simulink model "sldrtex_model"  (R2020a)
settings: Solver=FixedStepAuto  StartTime=0.0  StopTime=600  RelTol=1e-3  EnableMultiTasking=on
settings Model: Creator=Ben  LastModifiedBy=Ben
settings SolverCC: AutoInsertRateTranBlk=on
settings DataIOCC: SaveFormat=StructureWithTime
settings OptimizationCC: BlockReduction=off  OptimizeBlockIOStorage=off
settings RTWCC: Description=Simulink Desktop Real-Time  SystemTargetFile=sldrt.tlc  TemplateMakefile=sldrt.tmf  RTWCompilerOptimization=on
settings CodeAppCC: MaxIdLength=95
settings SimulinkDesktopRealTimeCC: TargetPreCompLibLocation=C:\Program Files\MATLAB\R2020a\toolbox\sldrt\lib\win64  TargetLangStandard=C89/C90 (ANSI)

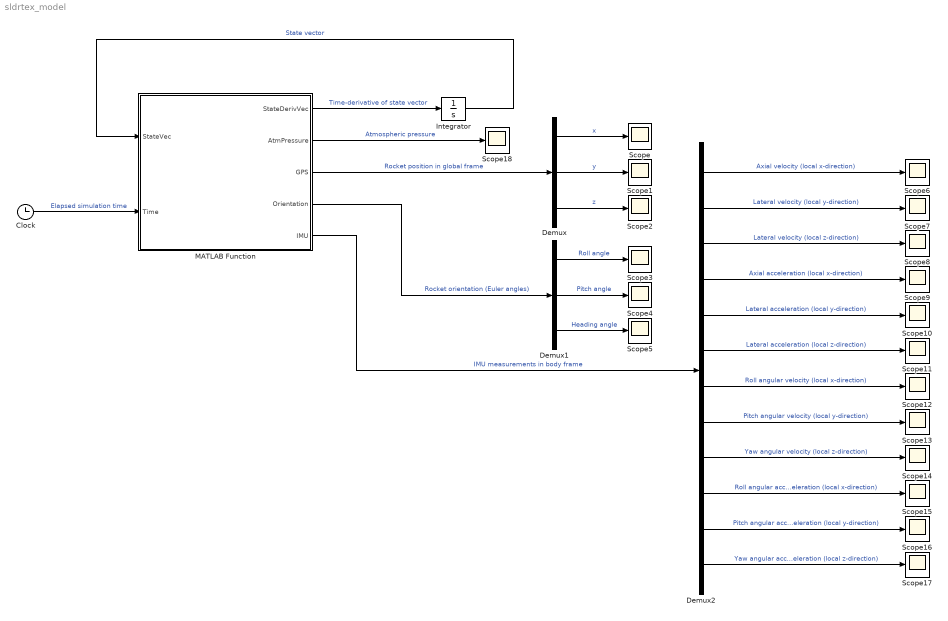
== system sldrtex_model ==
  Clock : Clock
  Demux : Demux  Outputs=3
  Demux1 : Demux  Outputs=3
  Demux2 : Demux  Outputs=12
  Integrator : Integrator  InitialCondition=[0 0 1401 0 -89 0 0 0 0 0 0 0]'
  MATLAB Function : MATLAB Function  TreatAsAtomicUnit=on
  Scope{,1..18} (19 alike) : Scope
  wires:
  Integrator/1 -> MATLAB Function/1(StateVec)  "State vector"
  MATLAB Function/1(StateDerivVec) -> Integrator/1  "Time-derivative of state vector"
  Clock/1 -> MATLAB Function/2(Time)  "Elapsed simulation time"
  MATLAB Function/2(AtmPressure) -> Scope18/1  "Atmospheric pressure"
  MATLAB Function/3(GPS) -> Demux/1  "Rocket position in global frame"
  MATLAB Function/4(Orientation) -> Demux1/1  "Rocket orientation (Euler angles)"
  MATLAB Function/5(IMU) -> Demux2/1  "IMU measurements in body frame"
  Demux/1 -> Scope/1  "x"
  Demux/2 -> Scope1/1  "y"
  Demux/3 -> Scope2/1  "z"
  Demux1/1 -> Scope3/1  "Roll angle"
  Demux1/3 -> Scope5/1  "Heading angle"
  Demux1/2 -> Scope4/1  "Pitch angle"
  Demux2/1 -> Scope6/1  "Axial velocity (local x-direction)"
  Demux2/2 -> Scope7/1  "Lateral velocity (local y-direction)"
  Demux2/3 -> Scope8/1  "Lateral velocity (local z-direction)"
  Demux2/4 -> Scope9/1  "Axial acceleration (local x-direction)"
  Demux2/7 -> Scope12/1  "Roll angular velocity (local x-direction)"
  Demux2/5 -> Scope10/1  "Lateral acceleration (local y-direction)"
  Demux2/8 -> Scope13/1  "Pitch angular velocity (local y-direction)"
  Demux2/6 -> Scope11/1  "Lateral acceleration (local z-direction)"
  Demux2/11 -> Scope16/1  "Pitch angular acceleration (local y-direction)"
  Demux2/9 -> Scope14/1  "Yaw angular velocity (local z-direction)"
  Demux2/12 -> Scope17/1  "Yaw angular acceleration (local z-direction)"
  Demux2/10 -> Scope15/1  "Roll angular acceleration (local x-direction)"

== matlab function sldrtex_model/MATLAB Function ==
  data: StateVec input double size=12,1; StateDerivVec output double size=12,1; Time input double size=1,1; AtmPressure output double size=1,1; GPS output double size=3,1; Orientation output double size=3,1; IMU output double size=12,1
function [StateDerivVec,AtmPressure,GPS,Orientation,IMU] = RocketDynModel_Sim(StateVec,Time)
%% Extract states and inputs
% States
PosVec = StateVec(1:3);
RollAngle = StateVec(4);
ElevAngle = StateVec(5);
HeadAngle = StateVec(6);
VelVec = StateVec(7:9);
AngVelVec_B = StateVec(10:12);

%% Define parameters
% Global properties
EarthRad = 6371.009e3;
GravAccelSL = 9.81;
WindVelVec = [0 0 0]';
SpHeatRatio = 1.4;

% Rocket physical properties
BurnTime = 34;
LoadMass = 711.9440829;
FuseDia = 0.508;
FuseLength = 7.90936;
PropFlowRate = 12.5;
NozzleEff = 0.98;
C_Star = 1580.684648;
ExitPressure = 78522.89615;
ChamberPressure = 950000;
ExpAreaRatio = 2.5;

% Rocket drag properties
P = load('Rocket drag data.mat');
MachNumData = P.RocketDragData(:,1);
DragCoeffData = P.RocketDragData(:,2);
DragArea = pi/4*FuseDia^2;
ACRelBasePosVec_B = [0.625 0 0]';
DirVec_B = [1 0 0]';

% Rocket launch properties
LaunchAngle = 89;
if Time <= 0
    if ElevAngle ~= -LaunchAngle
        error('Launch angle does not match initial elevation angle...');
    end
end
InitDistAlongRail = 0;
LaunchAlt = 1401;
RailLength = 15;
RailFricCoeff = 0;
LaunchVec = [
 cosd(LaunchAngle);
 0;
 sind(LaunchAngle)];

% Chute properties
BalluteAlt = 75000;
MainChuteAlt = 3000;
BalluteDragCoeff = 0.75;
MainChuteDragCoeff = 0.53;
BalluteLineLength = 5;
MainChuteLineLength = 7.148;
BalluteDia = 1;
MainChuteDia = 4.13;
NumBallutes = 3;
NumMainChutes = 3;
BalluteArea = NumBallutes*pi/4*(BalluteDia^2);
MainChuteArea = NumMainChutes*pi/4*(MainChuteDia^2);
ChuteRelBasePosVec_B = [5.66 0 0]';

% Rocket interial properties
Mass = ComputeRocketMass(Time,BurnTime,LoadMass,PropFlowRate);
[CGRelBasePosVec_B,CGRelBaseVelVec_B,CGRelBaseAccVec_B] =...
 ComputeCGRelBase(Time,BurnTime);
MOIMat = [ % Fix this to account for non-centered CG along cylinder
 (1/2)*Mass*(FuseDia/2)^2 0 0;
 0 (1/12)*Mass*(3*(FuseDia/2)^2 + FuseLength^2) 0;
 0 0 (1/12)*Mass*(3*(FuseDia/2)^2 + FuseLength^2)];
[AirDensity,SoundSpeed,~,AtmPressure,~,~,~] = atmos(PosVec(3),0,[],'SI','geometric',false);
GravAccel = GravAccelSL*((EarthRad/(EarthRad + PosVec(3)))^2);

%% Kinematics
% Fuselage rotation matrices
HeadRotMat = [
 cosd(HeadAngle) -sind(HeadAngle) 0;
 sind(HeadAngle) cosd(HeadAngle) 0;
 0 0 1];
ElevRotMat = [
 cosd(ElevAngle) 0 sind(ElevAngle);
 0 1 0;
 -sind(ElevAngle) 0 cosd(ElevAngle)];
RollRotMat = [
 1 0 0;
 0 cosd(RollAngle) -sind(RollAngle);
 0 sind(RollAngle) cosd(RollAngle)];
TotalRotMat = HeadRotMat*ElevRotMat*RollRotMat;

% Euler angle matrices
EulerRotMat = [
 1 0 -sind(ElevAngle);
 0 cosd(RollAngle) cosd(ElevAngle)*sind(RollAngle);
 0 -sind(RollAngle) cosd(ElevAngle)*cosd(RollAngle)];

% Forward coordinate transformation matrices
HeadTransMat_F = HeadRotMat';
ElevTransMat_F = ElevRotMat';
RollTransMat_F = RollRotMat';
TotalTransMat_F = RollTransMat_F*ElevTransMat_F*HeadTransMat_F;

% Backward coordinate transformation matrices
HeadTransMat_B = HeadRotMat;
ElevTransMat_B = ElevRotMat;
RollTransMat_B = RollRotMat;
TotalTransMat_B = HeadTransMat_B*ElevTransMat_B*RollTransMat_B;

% Rocket direction vector
DirVec = TotalRotMat*DirVec_B;

% Aerodynamic center velocity vector
ACVelVec =...
 VelVec...
 + TotalTransMat_B*(...
 -CGRelBaseVelVec_B...
 + cross(AngVelVec_B,ACRelBasePosVec_B - CGRelBasePosVec_B));

% Chute attachment point velocity
ChuteVelVec =...
 VelVec...
 + TotalTransMat_B*(...
 -0*CGRelBaseVelVec_B...
 + cross(AngVelVec_B,ChuteRelBasePosVec_B - CGRelBasePosVec_B));

%% Check whether rocket has left launch rail
if PosVec(3) < RailLength*sind(LaunchAngle) + LaunchAlt
 %% Compute external forces
 % Thrust force
 ThrustForce = ComputeThrustMag(Time,BurnTime,NozzleEff,C_Star,ExitPressure,ChamberPressure,ExpAreaRatio,PropFlowRate,SpHeatRatio,GravAccelSL,AtmPressure);
 
 % Gravitational force
 GravForce = -Mass*GravAccel*sind(LaunchAngle);
 
 % Rail friction force
 FricForce = -RailFricCoeff*Mass*GravAccel*cosd(LaunchAngle);
 
 % Aerodynamic force
 DragForceVec = ComputeDragForceVec(ACVelVec,MachNumData,DragCoeffData,DragArea,WindVelVec,SoundSpeed,AirDensity);
 AeroForce = dot(DragForceVec,LaunchVec);
 
 % Net external force
 TotalForce = ThrustForce + GravForce + FricForce + AeroForce;
 
 %% Compute state derivatives
 AccVec = TotalForce/Mass*LaunchVec;
 AngAccVec_B = zeros(3,1);
else
 %% Kinetics - Forces
 % Gravitational force
 GravForceVec = [0 0 -Mass*GravAccel]';
 
 % Thrust force
 ThrustForce = ComputeThrustMag(Time,BurnTime,NozzleEff,C_Star,ExitPressure,ChamberPressure,ExpAreaRatio,PropFlowRate,SpHeatRatio,GravAccelSL,AtmPressure);
 ThrustForceVec = ThrustForce*DirVec;
 
 % Aerodynamic force
 DragForceVec = ComputeDragForceVec(ACVelVec,MachNumData,DragCoeffData,DragArea,WindVelVec,SoundSpeed,AirDensity);
 AeroForceVec = DragForceVec;
 
 % Ballute force (currently using massless parachute model)
 ChuteRelWindVelVec = WindVelVec - ChuteVelVec;
 if (VelVec(3) < 0) && (PosVec(3) < BalluteAlt) && (PosVec(3) > MainChuteAlt)
  BalluteForceVec =...
   0.5*BalluteDragCoeff*AirDensity*BalluteArea...
   *norm(ChuteRelWindVelVec)*ChuteRelWindVelVec;
 else
  BalluteForceVec = zeros(3,1);
 end
 
 % Main chute force (currently using massless parachute model)
 if (VelVec(3) < 0) && (PosVec(3) < MainChuteAlt)
  MainChuteForceVec =...
   0.5*MainChuteDragCoeff*AirDensity*MainChuteArea...
   *norm(ChuteRelWindVelVec)*ChuteRelWindVelVec;
 else
  MainChuteForceVec = zeros(3,1);
 end
 
 % Total force vector
 ForceVec =...
  GravForceVec + ThrustForceVec + AeroForceVec...
  + BalluteForceVec + MainChuteForceVec;
 
 %% Kinetics - Moments
 % Thrust damping moment
 if Time < BurnTime
  ThrustDampMomVec =...
   -PropFlowRate*cross(-CGRelBasePosVec_B,cross(AngVelVec_B,-CGRelBasePosVec_B));
 else
  ThrustDampMomVec = zeros(3,1);
 end
 
 % Fuselage aerodynamic moment
 AeroMomVec =...
  cross(ACRelBasePosVec_B - CGRelBasePosVec_B,TotalTransMat_F*AeroForceVec);
 
 % Ballute moment
 BalluteMomVec =...
  cross(ChuteRelBasePosVec_B - CGRelBasePosVec_B,TotalTransMat_F*BalluteForceVec);
 
 % Main chute moment
 MainChuteMomVec =...
  cross(ChuteRelBasePosVec_B - CGRelBasePosVec_B,TotalTransMat_F*MainChuteForceVec);
 
 % Total aerodynamic moment
 MomVec =...
  AeroMomVec + BalluteMomVec + MainChuteMomVec + ThrustDampMomVec;
 
 %% Compute state derivatives
 AccVec = ForceVec/Mass;
 AngAccVec_B = MOIMat\(...
  MomVec - cross(AngVelVec_B,MOIMat*AngVelVec_B));
end

%% Compile state derivative vector
StateDerivVec = [
 VelVec;
 EulerRotMat\AngVelVec_B;
 AccVec;
 AngAccVec_B];
% include time varying MOI effects in Euler's equation of motion

%% Measurements
% Define point along rocket where measurements are taken
% Define location relative to the base in the body frame
MeasPointPosRelBase = [0 0 0]';

% Measurement point position in global frame
GPS =...
 PosVec...
 + TotalTransMat_B*(MeasPointPosRelBase - CGRelBasePosVec_B);
% GPS = GPS';

% Atmospheric pressure
[~,~,~,AtmPressure,~,~,~] = atmos(GPS(3),0,[],'SI','geometric',false);

% Rocket orientation (Euler angles)
Orientation = [
 RollAngle;
 ElevAngle;
 HeadAngle];
% Orientation = Orientation';

% Initialize IMU data vector
IMU = zeros(12,1);

% Measurement point velocity in body frame
IMU(1:3) =...
 TotalTransMat_F*VelVec - CGRelBaseVelVec_B...
 + cross(AngVelVec_B,MeasPointPosRelBase - CGRelBasePosVec_B);

% Measurement point acceleration in body frame
IMU(4:6) =...
 TotalTransMat_F*AccVec - CGRelBaseAccVec_B...
 - 2*cross(AngVelVec_B,CGRelBaseVelVec_B)...
 + cross(AngAccVec_B,MeasPointPosRelBase - CGRelBasePosVec_B)...
  + cross(AngAccVec_B,cross(AngAccVec_B,MeasPointPosRelBase - CGRelBasePosVec_B));

% Angular velocity in body frame
IMU(7:9) = AngVelVec_B;

% Angular acceleration in body frame
IMU(10:12) = AngAccVec_B;
% IMU = IMU';
